simulink model "Sensor_Fusion_Kalman_Filter"  (R2017a)
settings: Solver=FixedStepDiscrete  StartTime=0.0  StopTime=inf  FixedStep=0.001  RelTol=1e-3  EnableMultiTasking=on
libraries: instrumentlib x1
settings Model: Creator=Roger  LastModifiedBy=Roger
settings DataIOCC: LimitDataPoints=on  SaveFormat=Array
settings OptimizationCC: LifeSpan=inf
settings DebuggingCC: SFUnexpectedBacktrackingDiag=warning  SFNoUnconditionalDefaultTransitionDiag=warning  SFExecutionAtInitializationDiag=none
settings HardwareCC: ProdBitPerPointer=32  ProdBitPerSizeT=32  ProdBitPerPtrDiffT=32  ProdLargestAtomicFloat=None  ProdIntDivRoundTo=Undefined  ProdEndianess=Unspecified  ProdWordSize=32  ProdHWDeviceType=32-bit Generic
settings ModelReferenceCC: PropagateSignalLabelsOutOfModel=off
settings GRTTargetCC: TargetLangStandard=C89/C90 (ANSI)  GeneratePreprocessorConditionals=Disable all
settings ConfigComp: CovMetricSettings=dw  CovHtmlReporting=on  CovSaveCumulativeToWorkspaceVar=on  CovSaveSingleToWorkspaceVar=on  CovExternalEMLEnable=off

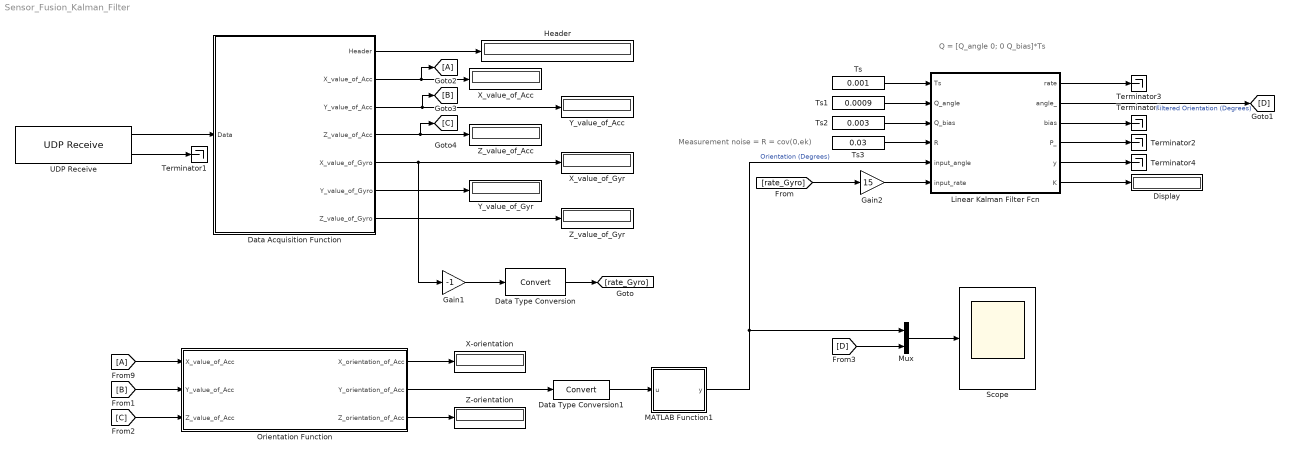
== system Sensor_Fusion_Kalman_Filter ==
  note: Measurement noise = R = cov(0,ek)
  note: Q = [Q_angle 0; 0 Q_bias]*Ts
  Data Acquisition Function : MATLAB Function  TreatAsAtomicUnit=on
  Data Type Conversion : DataTypeConversion
  Data Type Conversion1 : DataTypeConversion
  Display : Display
  Gain1 : Gain  Gain=-1
  Gain2 : Gain  Gain=15
  Header : Display
  Linear Kalman Filter Fcn : MATLAB Function  TreatAsAtomicUnit=on
  MATLAB Function1 : MATLAB Function  TreatAsAtomicUnit=on
  Mux : Mux  Inputs=2
  Orientation Function : MATLAB Function  TreatAsAtomicUnit=on
  Scope : Scope
  Terminator{1..5} (5 alike) : Terminator
  Ts : Constant  Value=0.001
  Ts1 : Constant  Value=0.0009
  Ts2 : Constant  Value=0.003
  Ts3 : Constant  Value=0.03
  UDP Receive : instrumentlib/UDP Receive  Priority=3  Host=172.20.10.1  Port=61422  LocalPort=58783  DataSize="[1  111]"  EnableBlockingMode=off  Timeout=10  SampleTime=0.001  DataType=uint8  ByteOrder=LittleEndian
      settings: SourceProductName=Instrument Control Toolbox
  X-orientation : Display
      settings: Format=bank
  X_value_of_Acc : Display
      settings: Format=bank
  X_value_of_Gyr : Display
      settings: Format=bank
  Y_value_of_Acc : Display
      settings: Format=bank
  Y_value_of_Gyr : Display
      settings: Format=bank
  Z-orientation : Display
      settings: Format=bank
  Z_value_of_Acc : Display
      settings: Format=bank
  Z_value_of_Gyr : Display
      settings: Format=bank
  wires:
  UDP Receive/1 -> Data Acquisition Function/1(Data)
  Data Acquisition Function/1(Header) -> Header/1
  Orientation Function/1(X_orientation_of_Acc) -> X-orientation/1
  [A] -> Orientation Function/1(X_value_of_Acc)
  Gain1/1 -> Data Type Conversion/1
  UDP Receive/2 -> Terminator1/1
  Data Type Conversion1/1 -> MATLAB Function1/1(u)
  Data Type Conversion/1 -> [rate_Gyro]
  [rate_Gyro] -> Gain2/1
  Orientation Function/2(Y_orientation_of_Acc) -> Data Type Conversion1/1
  Data Acquisition Function/2(X_value_of_Acc) -> [A], X_value_of_Acc/1
  Data Acquisition Function/3(Y_value_of_Acc) -> [B], Y_value_of_Acc/1
  Data Acquisition Function/7(Z_value_of_Gyro) -> Z_value_of_Gyr/1
  Data Acquisition Function/6(Y_value_of_Gyro) -> Y_value_of_Gyr/1
  Data Acquisition Function/5(X_value_of_Gyro) -> Gain1/1, X_value_of_Gyr/1
  Data Acquisition Function/4(Z_value_of_Acc) -> [C], Z_value_of_Acc/1
  Ts3/1 -> Linear Kalman Filter Fcn/4(R)
  Ts/1 -> Linear Kalman Filter Fcn/1(Ts)
  Ts1/1 -> Linear Kalman Filter Fcn/2(Q_angle)
  Ts2/1 -> Linear Kalman Filter Fcn/3(Q_bias)
  Gain2/1 -> Linear Kalman Filter Fcn/6(input_rate)
  Orientation Function/3(Z_orientation_of_Acc) -> Z-orientation/1
  [B] -> Orientation Function/2(Y_value_of_Acc)
  [C] -> Orientation Function/3(Z_value_of_Acc)
  Linear Kalman Filter Fcn/5(y) -> Terminator4/1
  Linear Kalman Filter Fcn/4(P_) -> Terminator2/1
  Linear Kalman Filter Fcn/3(bias) -> Terminator5/1
  Linear Kalman Filter Fcn/1(rate) -> Terminator3/1
  Linear Kalman Filter Fcn/6(K) -> Display/1
  Mux/1 -> Scope/1
  Linear Kalman Filter Fcn/2(angle_) -> [D]  "Filtered Orientation (Degrees)"
  [D] -> Mux/2
  MATLAB Function1/1(y) -> Mux/1, Linear Kalman Filter Fcn/5(input_angle)  "Orientation (Degrees)"

== matlab function Sensor_Fusion_Kalman_Filter/Data Acquisition Function ==
  data: Data input; Header output; X_value_of_Acc output single size=1 [-1000..1000]; Y_value_of_Acc output single size=1 [-1000..1000]; Z_value_of_Acc output single size=1 [-1000000..1000000]; X_value_of_Gyro output single size=1 [-1000..1000]; Y_value_of_Gyro output single size=1 [-1000..1000]; Z_value_of_Gyro output single size=1 [-1000..1000]
% Reading IMU packet bytes from Sensor Stream App 
% Author: RM van Rensburg
% Date: 26-04-2015
% Version: 1.0, tested on Matlab R2015a

function [Header,...
          X_value_of_Acc,Y_value_of_Acc, Z_value_of_Acc,...
          X_value_of_Gyro, Y_value_of_Gyro, Z_value_of_Gyro]...
          = fcn(Data)
             
% Header packet
Header = Data(1:4);

% Accelerometer data
X_value_of_Acc = typecast(uint8(Data(5:8)),'single');
Y_value_of_Acc = typecast(uint8(Data(9:12)),'single');
Z_value_of_Acc = typecast(uint8(Data(13:16)),'single');

% Gyroscope data
X_value_of_Gyro = typecast(uint8(Data(17:20)),'single');
Y_value_of_Gyro = typecast(uint8(Data(21:24)),'single');
Z_value_of_Gyro = typecast(uint8(Data(25:28)),'single');

% Proximity sensor
% X_value_of_Tes = typecast(uint8(Data(29:36)),'double');
% Y_value_of_Tes = typecast(uint8(Data(37:44)),'double');
% Z_value_of_Tes = typecast(uint8(Data(45:52)),'double');

== matlab function Sensor_Fusion_Kalman_Filter/Orientation Function ==
  data: X_value_of_Acc input; X_orientation_of_Acc output; Y_orientation_of_Acc output; Z_orientation_of_Acc output; Y_value_of_Acc input; Z_value_of_Acc input
% Computing orientation of tri-axial acclerometer data from IMU 
% Author: RM van Rensburg
% Date: 26-04-2015
% Version: 1.0,tested on Matlab R2015a

function [X_orientation_of_Acc,...
          Y_orientation_of_Acc,...
          Z_orientation_of_Acc]...
          = OrientationFcn(X_value_of_Acc,Y_value_of_Acc,Z_value_of_Acc)
     
      
% Using x and y from accelerometer (g-forces), calculate x and y angles
% Data directly obtained from IMU
% Using the following formulae
% Ax = arctan{X/sqrt(Y*Y + Z*Z)}
% Ay = arctan{Y/sqrt(X*X + Z*Z)}

% Computing the X*X, Y*Y, Z*Z
X2 = power(X_value_of_Acc,2);
Y2 = power(Y_value_of_Acc,2);
Z2 = power(Z_value_of_Acc,2);

% x-axis angle
result = sqrt(Y2 + Z2);
result = X_value_of_Acc / result;
x_angle_rad = atan(result);
X_orientation_of_Acc = (x_angle_rad * 180) / pi;

% y-axis angle
result = sqrt(X2 + Z2);
result = Y_value_of_Acc / result;
y_angle_rad = atan(result);
Y_orientation_of_Acc = (y_angle_rad * 180) / pi;

% z-axis angle
result = sqrt(Y2 + X2);
result = Z_value_of_Acc / result;
z_angle_rad = atan(result);
Z_orientation_of_Acc = (z_angle_rad * 180) / pi;

end

== matlab function Sensor_Fusion_Kalman_Filter/MATLAB Function1 ==
  data: u input; y output
function y = fcn(u)

if(isnan(u))
y=0;
else
y=u;
end

== matlab function Sensor_Fusion_Kalman_Filter/Linear Kalman Filter Fcn ==
  data: Ts input; Q_angle input; Q_bias input; R input; input_angle input; rate output; input_rate input; angle_ output; bias output; P_ output; y output; K output
% Sensor fusion linear-Kalman filter
% Author: RM van Rensburg
% Date: 26-04-2015
% Version: 1.0, tested on Matlab R2015a

function [rate,angle_,bias,P_,y,K] = Kalmanf(Ts,...
                                             Q_angle,Q_bias,R,...
                                             input_angle,...
                                             input_rate)
                      
% Process noise covariance matrix  
Q = [Q_angle 0;0 Q_bias] * Ts;
A = [1  -Ts;0  1];
C = [1 0];
bias = 0.0;

rate = input_rate - bias;

persistent angle;
if isempty(angle)
    angle = 0;
else angle = angle + (Ts * rate); 
end
angle_= angle;
                    
persistent P;
if isempty(P)
    P = [0 0 ; 0 0]; 
else P = A*P*A' + Q;
end
P_=P;

% Estimate error 
S = C*P*C' + R; 
% Kalman gain
K = (P_*C')/S; 
% Angle difference 
y = input_angle - angle_; 
xk = angle_ + K*y;
angle_ = xk(1);
bias = xk(2);
angle = angle_;

% Update the error covariance 
I = [1 0;0 1];
P_ = (I - K*C)*P_;
% or
% Joseph form (more stable)
% P_ = (I - K*C)*P_*(I - K*C) + K*R*K';
P = P_;

return

end
